simulink model "Magnet2V8"  (R2020a)
settings: Solver=FixedStepAuto  StartTime=0.0  StopTime=1.5  FixedStep=deltat  RelTol=1e-3  EnableMultiTasking=on
InitFcn:
  | %load A.mat;
  | %A = A;
  | %load B.mat;
  | %B = Expression1;
  | %load C.mat;
  | %C = C;
  | %load D.mat;
  | %D = D;
  | 
  | %i = .01;
  | %Q = eye(3)*i;
  | %N = 0;
  | %j = 1000;
  | %R = zeros(1, 1)+j;
  | 
  | %load Ad.mat;
  | %Ad = Ad;
  | %load Bd.mat;
  | %Bd = Bd;
  | %load Cd.mat;
  | %Cd = Cd;
  | %load Dd.mat;
  | %Dd = Dd;
  | 
  | run('script1.m');
  | %Q = eye(3)*0;
  | %R = 5e-07;
  | %N = 0;
  | %MeasurementOffset = .095;
undefined symbols (not defined in the file): Ad, Bd, Cd, Dd, deltat, DiscIntNeverNeededParam, Discrete, Kdlqr, Krd, MeasurementOffset, N, Q, R, Time
libraries: simulink x5, vrlib x2, ctrlSharedLib x1, eeGeneralControl x1
settings Model: Creator=bernardohasbach  LastModifiedBy=josh
settings SolverCC: AlgebraicLoopSolver=LineSearch  AutoInsertRateTranBlk=on
settings DataIOCC: SaveState=on
settings OptimizationCC: PassReuseOutputArgsAs=Individual arguments  OptimizeBlockOrder=speed  DifferentSizesBufferReuse=on  EfficientTunableParamExpr=on
settings DebuggingCC: ParameterTunabilityLossMsg=error
settings HardwareCC: TargetBitPerLong=64  TargetBitPerPointer=64  TargetBitPerSizeT=64  TargetBitPerPtrDiffT=64  TargetLongLongMode=on  TargetIntDivRoundTo=Zero  TargetEndianess=LittleEndian  TargetWordSize=64  TargetHWDeviceType=MATLAB Host  ProdEqTarget=off
settings SFSimCC: MATLABDynamicMemAlloc=off
settings RTWCC: Description=Embedded Coder (host-based shared library target)  SystemTargetFile=ert_shrlib.tlc  TemplateMakefile=ert_default_tmf  RTWVerbose=off  CustomDefine=-DTHIS_MODEL_NAME=$(PRODUCT_NAME)  BuildConfiguration=Faster Runs  IncludeHyperlinkInReport=on
settings RTWCC: CustomSourceCode=|
  | #define CONCAT(str1, str2, str3) CONCAT_(str1, str2, str3)
  | #define CONCAT_(str1, str2, str3) str1 ## str2 ## str3
  | #define GET_MMI_FUNC    CONCAT(THIS_MODEL_NAME, _GetCAPImmi    ,   )
  | #define RT_MODEL_STRUCT CONCAT(RT_MODEL_      , THIS_MODEL_NAME, _T)
  | 
  | void* GET_MMI_FUNC(void* voidPtrToRealTimeStructure)
  | {
  |    rtwCAPI_ModelMappingInfo* mmiPtr = &(rtmGetDataMapInfo( ( RT_MODEL_STRUCT * )(voidPtrToRealTimeStructure) ).mmi);
  |    return (void*) mmiPtr;
  | }
settings CodeAppCC: ForceParamTrailComments=on  GenerateComments=off  IgnoreCustomStorageClasses=off  OperatorAnnotations=on  SimulinkDataObjDesc=on  SFDataObjDesc=on  InsertBlockDesc=on
settings STFCustomTargetCC: TargetLangStandard=C99 (ISO)  MultiwordLength=256  ParMdlRefBuildCompliant=on  CompOptLevelCompliant=on  IncludeMdlTerminateFcn=off  CombineOutputUpdateFcns=on  CombineSignalStateStructs=on  ERTCustomFileBanners=on  SupportAbsoluteTime=off  MultiInstanceERTCode=on  CodeInterfacePackaging=Reusable function  SupportComplex=off  SupportNonInlinedSFcns=off  RemoveResetFunc=on  MATLABClassNameForMDSCustomization=Simulink.SoftwareTarget.ERTCustomization  ModelStepFunctionPrototypeControlCompliant=on  GenerateAllocFcn=on  UseToolchainInfoCompliant=on  SystemTargetFile=ert_shrlib.tlc
settings ERTTargetCC: TargetLangStandard=C99 (ISO)  ConcurrentExecutionCompliant=off  IncludeMdlTerminateFcn=off  CombineSignalStateStructs=on  SupportAbsoluteTime=off  MultiInstanceERTCode=on  CodeInterfacePackaging=Reusable function  SupportComplex=off  SupportContinuousTime=on  CPPClassGenCompliant=off  GenerateAllocFcn=on  RootIOFormat=Part of model data structure  RTWCAPIParams=on  RTWCAPIRootIO=on  ERTCustomFileTemplate=example_file_process.tlc

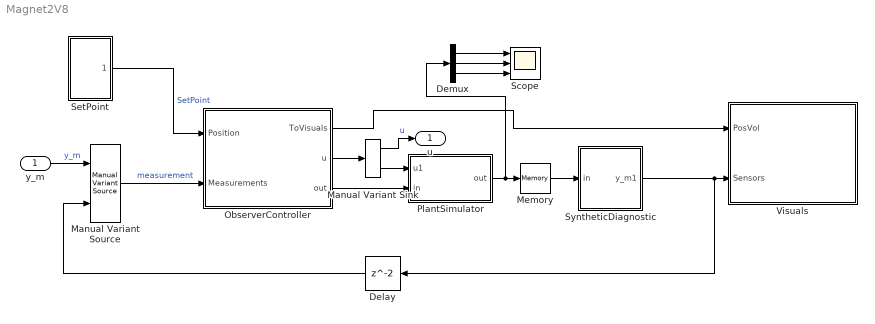
== system Magnet2V8 ==
  y_m : Inport
  Delay : Delay
  Demux : Demux  Outputs=3
  Manual Variant Sink : simulink/Signal Routing/Manual Variant Sink  NumChoices=2  LabelModeActiveChoice=V_2
  Manual Variant Source : simulink/Signal Routing/Manual Variant Source  NumChoices=2  LabelModeActiveChoice=V_2
  Memory : Memory  InheritSampleTime=on  LinearizeMemory=on  LinearizeAsDelay=on
  ObserverController : Subsystem  TreatAsAtomicUnit=on  SystemSampleTime=.01
  PlantSimulator : Subsystem  TreatAsAtomicUnit=on  SystemSampleTime=.01
  Scope : Scope  NumInputPorts=3
  SetPoint : Subsystem  TreatAsAtomicUnit=on  SystemSampleTime=.01
  SyntheticDiagnostic : Subsystem  TreatAsAtomicUnit=on  SystemSampleTime=.01
  Visuals : Subsystem
  u : Outport
  wires:
  ObserverController/1(ToVisuals) -> Visuals/1(PosVol)
  SyntheticDiagnostic/1(y_m1) -> Delay/1, Visuals/2(Sensors)
  ObserverController/2(u) -> Manual Variant Sink/1
  Manual Variant Sink/2 -> PlantSimulator/1(u1)
  Manual Variant Sink/1 -> u/1  "u"
  Manual Variant Source/1 -> ObserverController/2(Measurements)  "measurement"
  ObserverController/3(out) -> PlantSimulator/2(in)
  PlantSimulator/1(out) -> Demux/1, Memory/1
  Memory/1 -> SyntheticDiagnostic/1(in)
  y_m/1 -> Manual Variant Source/1  "y_m"
  SetPoint/1(SetPoint) -> ObserverController/1(Position)  "SetPoint"
  Demux/1 -> Scope/1
  Demux/2 -> Scope/2
  Demux/3 -> Scope/3
  Delay/1 -> Manual Variant Source/2

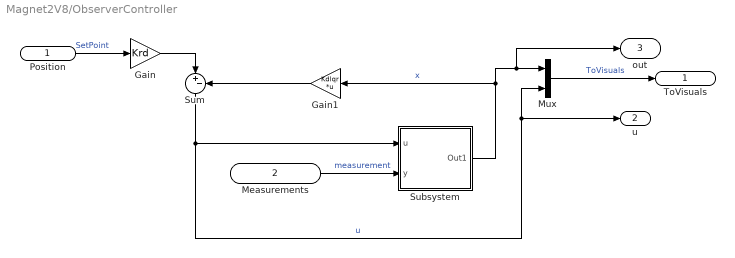
== system Magnet2V8/ObserverController ==
  Position : Inport  SampleTime=deltat
  Measurements : Inport  Port=2
  Gain : Gain  Gain=Krd
  Gain1 : Gain  Gain=Kdlqr  Multiplication=Matrix(K*u)
  Mux : Mux  Inputs=2
  Subsystem : Subsystem
  Sum : Sum  Inputs=|+-
  ToVisuals : Outport
  u : Outport  Port=2
  out : Outport  Port=3
  wires:
  Sum/1 -> u/1, Mux/2, Subsystem/1(u)  "u"
  Mux/1 -> ToVisuals/1  "ToVisuals"
  Gain1/1 -> Sum/2
  Measurements/1 -> Subsystem/2(y)  "measurement"
  Position/1 -> Gain/1  "SetPoint"
  Gain/1 -> Sum/1
  Subsystem/1(Out1) -> Mux/1, out/1, Gain1/1  "x"

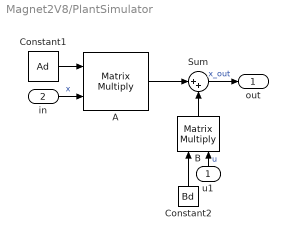
== system Magnet2V8/PlantSimulator ==
  u1 : Inport
  in : Inport  Port=2
  A : Product  Multiplication=Matrix(*)
  B : Product  Multiplication=Matrix(*)
  Constant1 : Constant  Value=Ad  SampleTime=deltat
  Constant2 : Constant  Value=Bd  SampleTime=deltat
  Sum : Sum  Inputs=|++
  out : Outport
  wires:
  B/1 -> Sum/2
  Sum/1 -> out/1  "x_out"
  A/1 -> Sum/1
  Constant2/1 -> B/1
  in/1 -> A/2  "x"
  u1/1 -> B/2  "u"
  Constant1/1 -> A/1

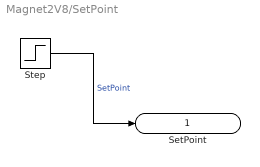
== system Magnet2V8/SetPoint ==
  Step : Step  After=.01  SampleTime=deltat
  SetPoint : Outport
  wires:
  Step/1 -> SetPoint/1  "SetPoint"

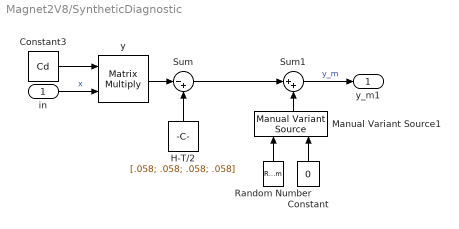
== system Magnet2V8/SyntheticDiagnostic ==
  in : Inport
  Constant : Constant  Value=0  SampleTime=deltat
  Constant3 : Constant  Value=Cd
  H-T/2 : Constant  Value=[.058; .058; .058; .058]  SampleTime=deltat
  Manual Variant Source1 : simulink/Signal Routing/Manual Variant Source  NumChoices=2  LabelModeActiveChoice=V_1
  Random Number : RandomNumber  Mean=[0;0;0;0]  Variance=[R;R;R;R]  Seed=[1;2;3;4]  SampleTime=deltat
  Sum : Sum  Inputs=|-+
  Sum1 : Sum  Inputs=|++
  y : Product  Multiplication=Matrix(*)
  y_m1 : Outport
  wires:
  Constant/1 -> Manual Variant Source1/2
  Manual Variant Source1/1 -> Sum1/2
  Constant3/1 -> y/1
  in/1 -> y/2  "x"
  Random Number/1 -> Manual Variant Source1/1
  Sum/1 -> Sum1/1
  Sum1/1 -> y_m1/1  "y_m"
  H-T/2/1 -> Sum/2
  y/1 -> Sum/1

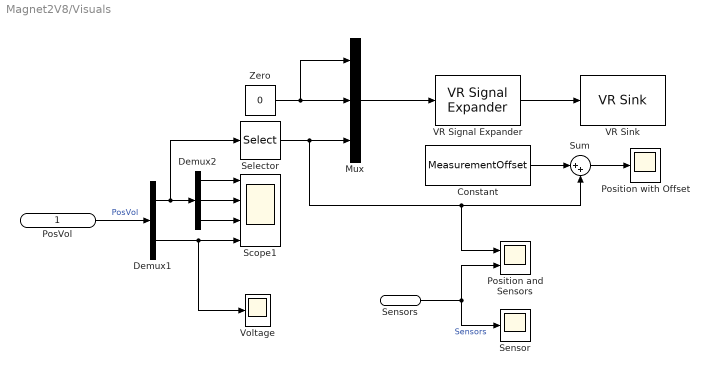
== system Magnet2V8/Visuals ==
  PosVol : Inport  SampleTime=deltat
  Sensors : Inport  Port=2
  Constant : Constant  Value=MeasurementOffset  SampleTime=deltat
  Demux1 : Demux  Outputs=2
  Demux2 : Demux  Outputs=3
  Mux : Mux  Inputs=3
  Position and Sensors : Scope  NumInputPorts=2
  Position with Offset : Scope
  Scope1 : Scope  NumInputPorts=4
  Selector : Selector  InputPortWidth=3  IndexOptions=Index vector (dialog)  Indices=[1]  OutputSizes=1
  Sensor : Scope
  Sum : Sum  Inputs=|++
  VR Signal Expander : vrlib/VR Signal Expander  outwidth=3  outidx=[1, 2, 3]
  VR Sink : vrlib/VR Sink  InstantiateOnLoad=on  SampleTime=0.1  ViewEnable=on  RemoteChange=off  RemoteView=off  FieldsWritten=Magnet.translation.3.1.1.double  WorldFileName=aparatusV3.x3d  AutoView=off  VideoDimensions=[]  AllowVariableSize=off
  Voltage : Scope
  Zero : Constant  Value=0  OutDataTypeStr=Inherit: Inherit via back propagation  SampleTime=deltat
  wires:
  Mux/1 -> VR Signal Expander/1
  VR Signal Expander/1 -> VR Sink/1
  Zero/1 -> Mux/1, Mux/2
  Sensors/1 -> Sensor/1, Position and Sensors/2  "Sensors"
  Selector/1 -> Position and Sensors/1, Sum/2, Mux/3
  Demux1/2 -> Scope1/4, Voltage/1
  PosVol/1 -> Demux1/1  "PosVol"
  Demux1/1 -> Selector/1, Demux2/1
  Demux2/3 -> Scope1/3
  Demux2/2 -> Scope1/2
  Demux2/1 -> Scope1/1
  Sum/1 -> Position with Offset/1
  Constant/1 -> Sum/1

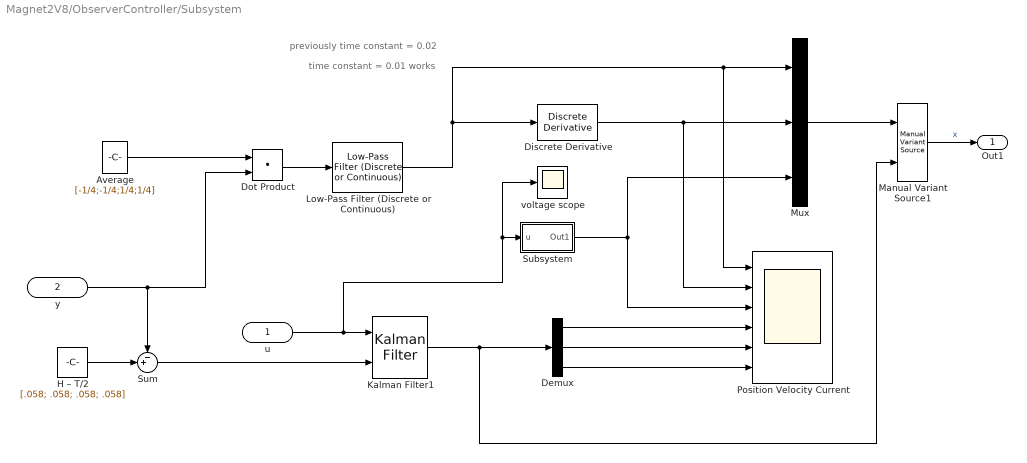
== system Magnet2V8/ObserverController/Subsystem ==
  note: previously time constant = 0.02
  note: time constant = 0.01 works
  u : Inport  SampleTime=deltat
  y : Inport  Port=2  SampleTime=deltat
  Average : Constant  Value=[-1/4;-1/4;1/4;1/4]
  Demux : Demux  Outputs=3
  Discrete Derivative : simulink/Discrete/Discrete Derivative  gainval=1.0  ICPrevScaledInput=0.0  OutMin=[]  OutMax=[]  OutDataType=fixdt(1, 16)  OutScaling=2^-10  DoSatur=off
  Dot Product : DotProduct  InputSameDT=on  OutDataTypeStr=Inherit: Inherit via internal rule
  H – T/2 : Constant  Value=[.058; .058; .058; .058]  SampleTime=deltat
  Kalman Filter1 : ctrlSharedLib/Kalman Filter  TimeDomain=Discrete-Time  UseCurrentEstimator=on  ModelSource=Individual A, B, C, D matrices  ModelSourceVariable=ss(0.95,1,1,0,1)  A=Ad  B=Bd  C=Cd  D=Dd  NumberOfStates=1  NumberOfInputs=1  NumberOfOutputs=1  InitialEstimateSource=Dialog  X0=0  P0=10  UseK=off  UseGH=off  NumberOfProcessNoiseInputs=1  G=1  TimeInvariantG=on  H=0  TimeInvariantH=on  Q=[Q;Q;Q]  TimeInvariantQ=on  R=[R;R;R;R]  TimeInvariantR=on  N=N  TimeInvariantN=on  AddInputPort=on  AddEnablePort=off  OutputEstimatedY=off  OutputP=off  Ts=deltat
  Low-Pass Filter (Discrete or Continuous) : eeGeneralControl/Low-Pass Filter (Discrete or Continuous)  K=1  T=.01  B=inf  A=-inf  init_option=Inherited from block input  x0=0  Ts=deltat
  Manual Variant Source1 : simulink/Signal Routing/Manual Variant Source  NumChoices=2  LabelModeActiveChoice=V_2
  Mux : Mux  Inputs=3
  Position Velocity Current : Scope  NumInputPorts=6
  Subsystem : Subsystem
  Sum : Sum  Inputs=-+|
  voltage scope : Scope
  Out1 : Outport
  wires:
  y/1 -> Dot Product/2, Sum/1
  Dot Product/1 -> Low-Pass Filter (Discrete or Continuous)/1
  u/1 -> voltage scope/1, Subsystem/1(u), Kalman Filter1/1
  Subsystem/1(Out1) -> Position Velocity Current/3, Mux/3
  Discrete Derivative/1 -> Position Velocity Current/2, Mux/2
  Kalman Filter1/1 -> Manual Variant Source1/2, Demux/1
  Demux/1 -> Position Velocity Current/4
  Demux/2 -> Position Velocity Current/5
  Demux/3 -> Position Velocity Current/6
  Low-Pass Filter (Discrete or Continuous)/1 -> Discrete Derivative/1, Position Velocity Current/1, Mux/1
  Manual Variant Source1/1 -> Out1/1  "x"
  Mux/1 -> Manual Variant Source1/1
  H – T/2/1 -> Sum/2
  Sum/1 -> Kalman Filter1/2
  Average/1 -> Dot Product/1

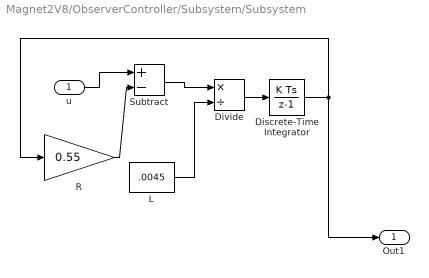
== system Magnet2V8/ObserverController/Subsystem/Subsystem ==
  u : Inport
  Discrete-Time Integrator : DiscreteIntegrator  SampleTime=deltat  ICPrevOutput=DiscIntNeverNeededParam  ICPrevScaledInput=DiscIntNeverNeededParam
  Divide : Product  Inputs=*/
  L : Constant  Value=.0045  SampleTime=deltat
  R : Gain  Gain=0.55
  Subtract : Sum  Inputs=+-
  Out1 : Outport
  wires:
  Discrete-Time Integrator/1 -> Out1/1, R/1
  Divide/1 -> Discrete-Time Integrator/1
  L/1 -> Divide/2
  Subtract/1 -> Divide/1
  R/1 -> Subtract/2
  u/1 -> Subtract/1
